simulink model "project"  (R2020a)
settings: Solver=VariableStepAuto  StartTime=0.0  StopTime=3  MaxStep=0.0001  RelTol=1e-3
model workspace (MATLAB code in the model file):
  | Pp=2;
  | Pc=4;
  | 
  | Rr=0.1023;
  | Rsp=0.0770;
  | Rsc=0.1023;
  | 
  | Lr=0.14302;
  | Lsp=0.08618;
  | Lsc=0.025913;
  | 
  | Lmp=0.0758;
  | Lmc=0.0733;
  | 
  | Ts=2e-5
libraries: powerlib_meascontrol x6, powerlib x1
settings Model: Creator=berthamafunu  LastModifiedBy=berthamafunu
settings SolverCC: AlgebraicLoopSolver=LineSearch
settings DebuggingCC: AlgebraicLoopMsg=none

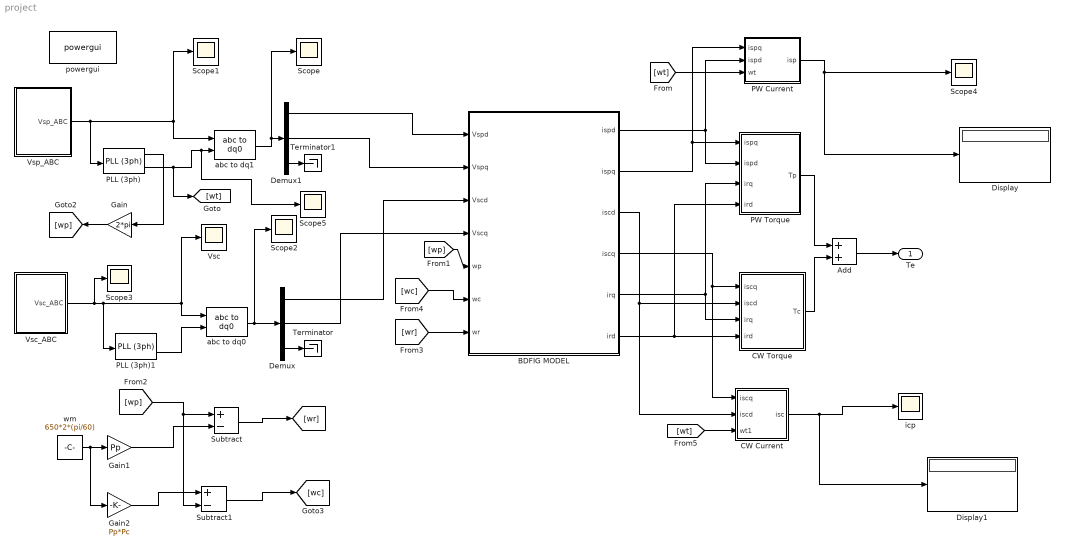
== system project ==
  Add : Sum
  BDFIG MODEL : Subsystem
  CW Current : Subsystem
  CW Torque : Subsystem
  Demux : Demux  Outputs=3
  Demux1 : Demux  Outputs=3
  Display : Display
  Display1 : Display
  Gain : Gain  Gain=2*pi
  Gain1 : Gain  Gain=Pp
  Gain2 : Gain  Gain=Pp*Pc
  PLL (3ph) : powerlib_meascontrol/PLL/PLL (3ph)  Fmin=45  Par_Init=[0, 50]  ParK=[212.93, 2267, 1]  TcD=Ts  MaxRateChangeFreq=12  FilterCutOffFreq=25  Ts=Ts  AGC=on
  PLL (3ph)1 : powerlib_meascontrol/PLL/PLL (3ph)  Fmin=45  Par_Init=[0, 50]  ParK=[212.93, 2267, 1]  TcD=Ts  MaxRateChangeFreq=12  FilterCutOffFreq=25  Ts=Ts  AGC=on
  PW Current : Subsystem
  "PW Torque " : Subsystem
  Scope{,1..5} (6 alike) : Scope
  Subtract : Sum  Inputs=+-
  Subtract1 : Sum  Inputs=+-
  Terminator : Terminator
  Terminator1 : Terminator
  Vsc : Scope
  Vsc_ABC : Subsystem
  Vsp_ABC : Subsystem
  abc to dq0 : powerlib_meascontrol/Transformations/abc to dq0  Alignment=90 degrees behind phase A axis
  abc to dq1 : powerlib_meascontrol/Transformations/abc to dq0  Alignment=90 degrees behind phase A axis
  icp : Scope
  powergui : powerlib/powergui  Priority=1  SimulationMode=Continuous  SampleTime=Ts  frequency=60  Iterations=50  frequencyindice=60  Pbase=100e6  ErrMax=1e-4  UnitsV=kV  UnitsW=MW  buscounter=0  FunctionMessages=off  echomessages=off  EnableUseOfTLC=off  CurrentSourceSwitches=off  DisableSnubberDevices=off  DisableRonSwitches=off  DisableVfSwitches=off  DisplayEquations=off  AutomaticDiscreteSolvers=off  SolverType=Tustin/Backward Euler (TBE)  Interpol=off  ExternalGateDelay=off  methode=off  Ts=100  x0status=blocks  SPID=on  SwTol=0  HookPort=off  NonlinearTolerance=1e-4  nMaxIteration=100  ContinueOnMaxIteration=off  RestoreLinks=warning  ResistiveCurrentMeasurement=off  Frange=[0:2:500]  Ylog=off  Xlog=on  ShowGrid=off  save=off  variable=ZData  structure=0  ZoomFFT=off  StartTime=0.0  cycles=1  DisplayStyle=1  fundamental=60  FreqAxis=off  MaxFrequency=1000  frequencyindicesteady=1  RmsSteady=1  display=off
  wm : Constant  Value=650*2*(pi/60)
  Te : Outport
  wires:
  BDFIG MODEL/2(ispq) -> PW Current/1(ispq), "PW Torque "/1(ispq)
  BDFIG MODEL/1(ispd) -> "PW Torque "/2(ispd), PW Current/2(ispd)
  BDFIG MODEL/6(ird) -> "PW Torque "/4(ird), CW Torque/4(ird)
  BDFIG MODEL/4(iscq) -> CW Current/1(iscq), CW Torque/1(iscq)
  BDFIG MODEL/3(iscd) -> CW Torque/2(iscd), CW Current/2(iscd)
  Demux/3 -> Terminator/1
  abc to dq0/1 -> Scope2/1, Demux/1
  abc to dq1/1 -> Scope/1, Demux1/1
  Demux1/3 -> Terminator1/1
  BDFIG MODEL/5(irq) -> "PW Torque "/3(irq), CW Torque/3(irq)
  "PW Torque "/1(Tp) -> Add/1
  CW Torque/1(Tc) -> Add/2
  Add/1 -> Te/1
  Vsp_ABC/1(Vsp_ABC) -> PLL (3ph)/1, Scope1/1, abc to dq1/1
  Vsc_ABC/1(Vsc_ABC) -> Scope3/1, PLL (3ph)1/1, abc to dq0/1, Vsc/1
  PLL (3ph)/2 -> Scope5/1, abc to dq1/2, [wt]
  Demux1/1 -> BDFIG MODEL/1(Vspd)
  Demux1/2 -> BDFIG MODEL/2(Vspq)
  Demux/1 -> BDFIG MODEL/3(Vscd)
  Demux/2 -> BDFIG MODEL/4(Vscq)
  [wt] -> PW Current/3(wt)
  PLL (3ph)/1 -> Gain/1
  Gain/1 -> [wp]
  [wp] -> BDFIG MODEL/5(wp)
  [wp] -> Subtract1/2, Subtract/1
  wm/1 -> Gain2/1, Gain1/1
  Gain1/1 -> Subtract/2
  Subtract/1 -> [wr]
  [wr] -> BDFIG MODEL/7(wr)
  PLL (3ph)1/2 -> abc to dq0/2
  Gain2/1 -> Subtract1/1
  Subtract1/1 -> [wc]
  [wc] -> BDFIG MODEL/6(wc)
  [wt] -> CW Current/3(wt1)
  PW Current/1(isp) -> Display/1, Scope4/1
  CW Current/1(isc) -> Display1/1, icp/1

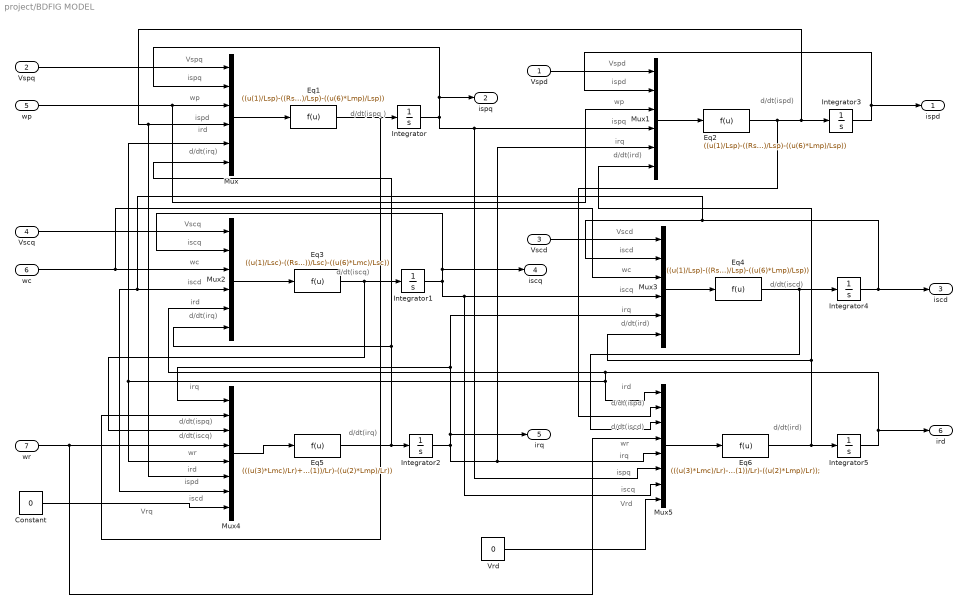
== system project/BDFIG MODEL ==
  note: Vrd
  note: Vrq
  note: d/dt(ird)
  note: d/dt(irq)
  note: d/dt(iscd)
  note: d/dt(iscq)
  note: d/dt(ispd)
  note: d/dt(ispq )
  note: ispd
  note: wr
  note: d/dt(irq)
  note: ird
  note: ispd
  note: wp
  note: ispq
  note: Vspq
  note: d/dt(ird)
  note: irq
  note: ispq
  note: wp
  note: ispd
  note: Vspd
  note: d/dt(irq)
  note: ird
  note: iscd
  note: wc
  note: iscq
  note: Vscq
  note: d/dt(ird)
  note: irq
  note: iscq
  note: wc
  note: iscd
  note: Vscd
  note: iscd
  note: ird
  note: d/dt(iscq)
  note: d/dt(ispq)
  note: irq
  note: ispq
  note: wr
  note: iscq
  note: irq
  note: d/dt(iscd)
  note: d/dt(ispd)
  note: ird
  Vspd : Inport
  Vspq : Inport  Port=2
  Vscd : Inport  Port=3
  Vscq : Inport  Port=4
  wp : Inport  Port=5
  wc : Inport  Port=6
  wr : Inport  Port=7
  Constant : Constant  Value=0
  Eq1 : Fcn  Expr=((u(1)/Lsp)-((Rsp*u(2))/Lsp)-(u(3)*u(4))-((u(3)*Lmp*u(5))/Lsp)-((u(6)*Lmp)/Lsp))
  Eq2 : Fcn  Expr=((u(1)/Lsp)-((Rsp*u(2))/Lsp)-(u(3)*u(4))+((u(3)*Lmp*u(5))/Lsp)-((u(6)*Lmp)/Lsp))
  Eq3 : Fcn  Expr=((u(1)/Lsc)-((Rsc*u(2))/Lsc)-(u(3)*u(4))+((u(3)*Lmc*u(5))/Lsc)-((u(6)*Lmc)/Lsc))
  Eq4 : Fcn  Expr=((u(1)/Lsp)-((Rsc*u(2))/Lsp)-(u(3)*u(4))+((u(3)*Lmp*u(5))/Lsp)-((u(6)*Lmp)/Lsp))
  Eq5 : Fcn  Expr=(((u(3)*Lmc)/Lr)+(u(4)*u(5))-((u(4)*Lmp*u(6))/Lr)+((u(4)*Lmc*u(7))/Lr)-((Rr*u(1))/Lr)-((u(2)*Lmp)/Lr))
  Eq6 : Fcn  Expr=(((u(3)*Lmc)/Lr)-(u(4)*u(5))-((u(4)*Lmp*u(6))/Lr)+((u(4)*Lmc*u(7))/Lr)-((Rr*u(1))/Lr)-((u(2)*Lmp)/Lr));
  Integrator{,1..5} (6 alike) : Integrator
  Mux{,1..3} (4 alike) : Mux  Inputs=6
  Mux4 : Mux  Inputs=8
  Mux5 : Mux  Inputs=8
  Vrd : Constant  Value=0
  ispd : Outport
  ispq : Outport  Port=2
  iscd : Outport  Port=3
  iscq : Outport  Port=4
  irq : Outport  Port=5
  ird : Outport  Port=6
  wires:
  Mux5/1 -> Eq6/1
  Mux2/1 -> Eq3/1
  Vscd/1 -> Mux3/1
  Eq3/1 -> Mux4/3, Integrator1/1
  Vspq/1 -> Mux/1
  Eq6/1 -> Mux1/6, Mux3/6, Integrator5/1
  Vrd/1 -> Mux5/8
  Integrator4/1 -> iscd/1, Mux4/7, Mux2/4, Mux3/2
  Constant/1 -> Mux4/8
  wr/1 -> Mux4/4, Mux5/4
  wc/1 -> Mux3/3, Mux2/3
  Integrator/1 -> Mux5/6, Mux1/4, ispq/1, Mux/2
  Eq5/1 -> Mux2/6, Mux/6, Integrator2/1
  Eq1/1 -> Mux4/2, Integrator/1
  wp/1 -> Mux1/3, Mux/3
  Integrator1/1 -> iscq/1, Mux2/2, Mux5/7, Mux3/4
  Integrator2/1 -> irq/1, Mux3/5, Mux4/1, Mux5/5, Mux1/5
  Vscq/1 -> Mux2/1
  Mux1/1 -> Eq2/1
  Eq2/1 -> Mux5/2, Mux4/6, Mux/4, Integrator3/1
  Eq4/1 -> Mux5/3, Integrator4/1
  Mux4/1 -> Eq5/1
  Mux/1 -> Eq1/1
  Vspd/1 -> Mux1/1
  Integrator5/1 -> ird/1, Mux2/5, Mux5/1, Mux/5, Mux4/5
  Mux3/1 -> Eq4/1
  Integrator3/1 -> ispd/1, Mux1/2

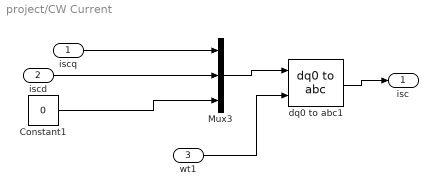
== system project/CW Current ==
  iscq : Inport
  iscd : Inport  Port=2
  wt1 : Inport  Port=3
  Constant1 : Constant  Value=0
  Mux3 : Mux  Inputs=3
  dq0 to abc1 : powerlib_meascontrol/Transformations/dq0 to abc  Alignment=90 degrees behind phase A axis
  isc : Outport
  wires:
  wt1/1 -> dq0 to abc1/2
  Constant1/1 -> Mux3/3
  iscd/1 -> Mux3/2
  dq0 to abc1/1 -> isc/1
  Mux3/1 -> dq0 to abc1/1
  iscq/1 -> Mux3/1

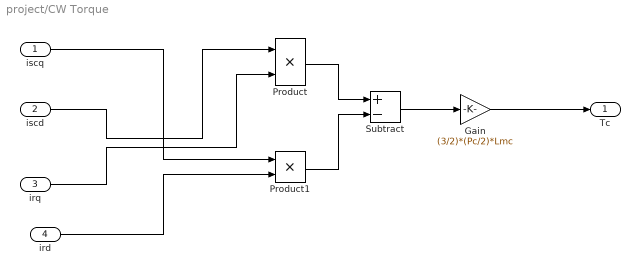
== system project/CW Torque ==
  iscq : Inport
  iscd : Inport  Port=2
  irq : Inport  Port=3
  ird : Inport  Port=4
  Gain : Gain  Gain=(3/2)*(Pc/2)*Lmc
  Product : Product
  Product1 : Product
  Subtract : Sum  Inputs=+-
  Tc : Outport
  wires:
  iscq/1 -> Product1/1
  iscd/1 -> Product/1
  Subtract/1 -> Gain/1
  Gain/1 -> Tc/1
  Product1/1 -> Subtract/2
  irq/1 -> Product/2
  Product/1 -> Subtract/1
  ird/1 -> Product1/2

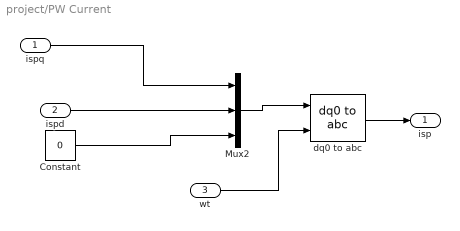
== system project/PW Current ==
  ispq : Inport
  ispd : Inport  Port=2
  wt : Inport  Port=3
  Constant : Constant  Value=0
  Mux2 : Mux  Inputs=3
  dq0 to abc : powerlib_meascontrol/Transformations/dq0 to abc  Alignment=90 degrees behind phase A axis
  isp : Outport
  wires:
  wt/1 -> dq0 to abc/2
  ispd/1 -> Mux2/2
  ispq/1 -> Mux2/1
  Mux2/1 -> dq0 to abc/1
  dq0 to abc/1 -> isp/1
  Constant/1 -> Mux2/3

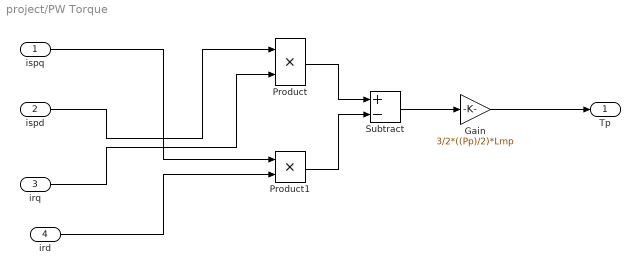
== system project/PW Torque  ==
  ispq : Inport
  ispd : Inport  Port=2
  irq : Inport  Port=3
  ird : Inport  Port=4
  Gain : Gain  Gain=3/2*((Pp)/2)*Lmp
  Product : Product
  Product1 : Product
  Subtract : Sum  Inputs=+-
  Tp : Outport
  wires:
  ird/1 -> Product1/2
  Product/1 -> Subtract/1
  irq/1 -> Product/2
  Product1/1 -> Subtract/2
  Gain/1 -> Tp/1
  Subtract/1 -> Gain/1
  ispd/1 -> Product/1
  ispq/1 -> Product1/1

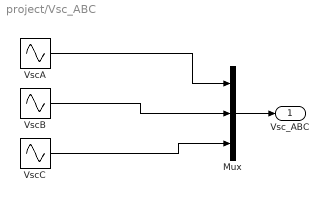
== system project/Vsc_ABC ==
  Mux : Mux  Inputs=3
  VscA : Sin  Amplitude=(178.02/sqrt(3))*sqrt(2)  Frequency=2*pi*50  SampleTime=Ts
  VscB : Sin  Amplitude=(178.02/sqrt(3))*sqrt(2)  Frequency=2*pi*50  Phase=-(2*pi)/3  SampleTime=Ts
  VscC : Sin  Amplitude=(178.02/sqrt(3))*sqrt(2)  Frequency=2*pi*50  Phase=(2*pi)/3  SampleTime=Ts
  Vsc_ABC : Outport
  wires:
  Mux/1 -> Vsc_ABC/1
  VscA/1 -> Mux/1
  VscB/1 -> Mux/2
  VscC/1 -> Mux/3

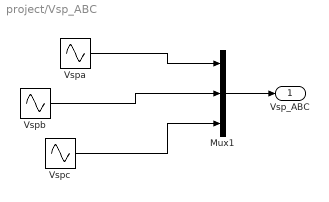
== system project/Vsp_ABC ==
  Mux1 : Mux  Inputs=3
  Vspa : Sin  Amplitude=0  Frequency=2*pi*50  SampleTime=Ts
  Vspb : Sin  Amplitude=0  Frequency=2*pi*50  Phase=-((2*pi)/3)  SampleTime=Ts
  Vspc : Sin  Amplitude=0  Frequency=2*pi*50  Phase=(2*pi)/3  SampleTime=Ts
  Vsp_ABC : Outport
  wires:
  Mux1/1 -> Vsp_ABC/1
  Vspb/1 -> Mux1/2
  Vspa/1 -> Mux1/1
  Vspc/1 -> Mux1/3
